simulink subsystem "Simulink_Model"  (R2022b)
settings: Solver=VariableStepAuto  StartTime=0.0  StopTime=10.0  RelTol=1e-3
model mask{pwr=0, Ra=0, La=0, Kphi=0, Be=0, Je=1e-8, Kg=0, enable_Tc=off, tau_c=0, enable_Tsb=off, tau_sb=0, w_sb=0, approximate=off, lambda=1}
  mask prompts: pwr "Vcc - Power Supply [V]:"; Ra "Ra - Armature Resitance [Ohm]:"; La "La - Armature Inductance [H]:"; Kphi "Kphi - Flux Constant [V*s]:"; Be "Be - Viscous Friction [N*m*s]:"; Je "Je - Inertia [Kg*m^2]:"; Kg "Kg - Gear ratio [#]:"; enable_Tc "Coulomb Friction"; tau_c "Tc - Static Friction [N*m]:"; enable_Tsb "Stribeck Friction"; tau_sb "Tsb - Breakaway Torque [N*m]:"; w_sb "w_sb - Breakaway Speed [rad/s]:"; approximate "Approximate sgn with tanh"; lambda "Sigmoid Exponent"
settings Model: Creator=gotta  LastModifiedBy=gotta

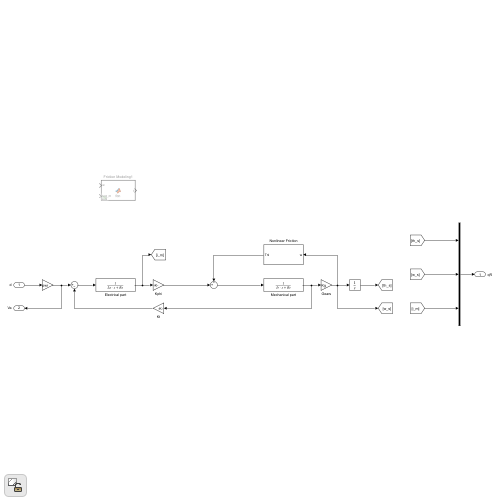
[thumbnail: Simulink's stored preview of the top-level diagram]
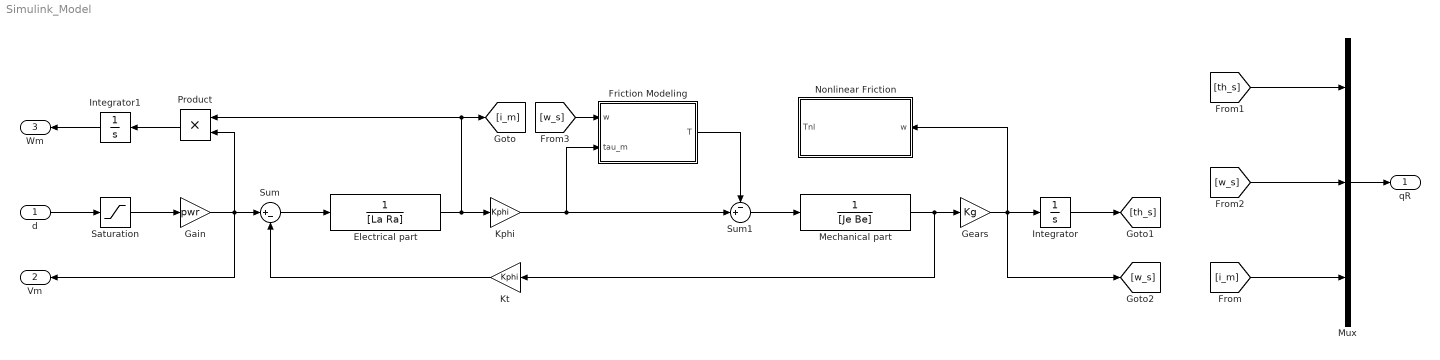
== system Simulink_Model ==
  d : Inport
  Electrical part : TransferFcn  Denominator=[La Ra]
  Friction Modeling : MATLAB Function  TreatAsAtomicUnit=on
  Gain : Gain  Gain=pwr
  Gears : Gain  Gain=Kg
  Integrator : Integrator
  Integrator1 : Integrator
  Kphi : Gain  Gain=Kphi
  Kt : Gain  Gain=Kphi
  Mechanical part : TransferFcn  Denominator=[Je Be]
  Mux : Mux  Inputs=3
  Nonlinear Friction : Subsystem
  Product : Product
  Saturation : Saturate  UpperLimit=1  LowerLimit=-1
  Sum : Sum  Inputs=|+-
  Sum1 : Sum  Inputs=-+|
  qR : Outport
  Vm : Outport  Port=2
  Wm : Outport  Port=3
  wires:
  [th_s] -> Mux/1
  [i_m] -> Mux/3
  [w_s] -> Mux/2
  Mux/1 -> qR/1
  Gain/1 -> Sum/1, Product/2, Vm/1
  Electrical part/1 -> Kphi/1, [i_m], Product/1
  Integrator/1 -> [th_s]
  Gears/1 -> Integrator/1, [w_s], Nonlinear Friction/1(w)
  Kt/1 -> Sum/2
  d/1 -> Saturation/1
  Kphi/1 -> Friction Modeling/2(tau_m), Sum1/2
  Sum/1 -> Electrical part/1
  Mechanical part/1 -> Gears/1, Kt/1
  Sum1/1 -> Mechanical part/1
  Saturation/1 -> Gain/1
  Product/1 -> Integrator1/1
  Integrator1/1 -> Wm/1
  [w_s] -> Friction Modeling/1(w)
  Friction Modeling/1(T) -> Sum1/1

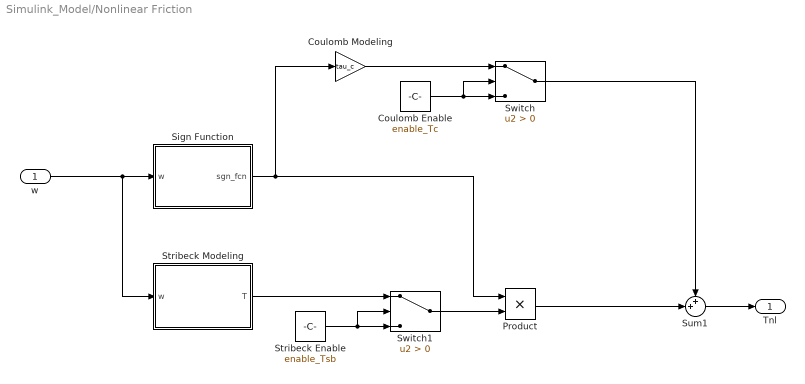
== system Simulink_Model/Nonlinear Friction ==
  w : Inport
  Coulomb Enable : Constant  Value=enable_Tc
  Coulomb Modeling : Gain  Gain=tau_c
  Product : Product
  Sign Function : MATLAB Function  TreatAsAtomicUnit=on
  Stribeck Enable : Constant  Value=enable_Tsb
  Stribeck Modeling : MATLAB Function  TreatAsAtomicUnit=on
  Sum1 : Sum  Inputs=++|
  Switch : Switch  Criteria=u2 > Threshold  SaturateOnIntegerOverflow=off  InputSameDT=off
  Switch1 : Switch  Criteria=u2 > Threshold  SaturateOnIntegerOverflow=off  InputSameDT=off
  Tnl : Outport
  wires:
  Product/1 -> Sum1/2
  Sign Function/1(sgn_fcn) -> Product/1, Coulomb Modeling/1
  Switch1/1 -> Product/2
  Stribeck Enable/1 -> Switch1/3, Switch1/2
  Coulomb Enable/1 -> Switch/3, Switch/2
  Coulomb Modeling/1 -> Switch/1
  Switch/1 -> Sum1/1
  Sum1/1 -> Tnl/1
  Stribeck Modeling/1(T) -> Switch1/1
  w/1 -> Sign Function/1(w), Stribeck Modeling/1(w)

== matlab function Simulink_Model/Friction Modeling ==
  data: w input; tau_m input; T output; tau_sb parameter; w_sb parameter; tau_c parameter; enable_Tc parameter; enable_Tsb parameter
function T = fcn(w, tau_m, tau_sb, w_sb, tau_c, enable_Tc, enable_Tsb)

T = 0; % linear model case

if (enable_Tc || enable_Tsb) 
    if abs(w) <= w_sb && abs(tau_m) <= tau_sb
        T = tau_m;
    else
        Tc = tau_c*sign(w)*enable_Tc;
        Tsb = (tau_sb - tau_c)*exp(-(w/w_sb)^2)*sign(w)*enable_Tsb;
        T = Tc + Tsb;
    end
end

== matlab function Simulink_Model/Nonlinear Friction/Sign Function ==
  data: w input; sgn_fcn output; approximate parameter; lambda parameter
function sgn_fcn = fcn(w, approximate, lambda)

% Sign function approximator
tan_sign = 2/(1+exp(-lambda*w)) - 1;

% Sign function selection
sgn_fcn = sign(w);
if approximate
    sgn_fcn = tan_sign;
end

== matlab function Simulink_Model/Nonlinear Friction/Stribeck Modeling ==
  data: w input; T output; tau_c parameter; tau_sb parameter; w_sb parameter
function T = fcn(w, tau_c, tau_sb, w_sb)


T = (tau_sb - tau_c)*exp(-(w / w_sb)^2);
